simulink model "robotarm_A12"  (R2018b)
settings: Solver=FixedStepAuto  StartTime=0.0  StopTime=options.T_train  RelTol=1e-3  AbsTol=1e-6
undefined symbols (not defined in the file or in its folder): options
libraries: neural x132, simulink x2
(part 4 of 6)

== system robotarm_A12/NN/Layer 3/Delays 1 ==
  "p{3}" : Inport  PortDimensions=30
      mask Display: e = 0.06;c1 = [120 230 180]/255;c2 = ([120 230 180]+0)/(256+128);c3 = ([120 230 180]+128)/(256+128);patch([0 1 1 0],[0 0 1 1],c1);patch([0 1 1 1-e 1-e 0+e],[0 0 1 1-e 0+e 0+e],c2);patch([0 0 1 1-e 0+e 0+e],[0 1 1 1-e 1-e 0+e],c3);plot([0 1 1 0 0],[0 0 1 1 0]);
  mux : Mux  Inputs=1
      mask Display: e = 0.06;c1 = [120 150 230]/255;c2 = ([120 150 230]+0)/383;c3 = ([120 150 230]+128)/383;patch([0 1 1 0],[0 0 1 1],c1);patch([0 1 1 1-e 1-e 0+e],[0 0 1 1-e 0+e 0+e],c2);patch([0 0 1 1-e 0+e 0+e],[0 1 1 1-e 1-e 0+e],c3);plot([0 1 1 0 0],[0 0 1 1 0]);disp('Mux')
  "pd{3,2}" : Outport
      mask Display: e = 0.06;c1 = [120 230 180]/255;c2 = ([120 230 180]+0)/(256+128);c3 = ([120 230 180]+128)/(256+128);patch([0 1 1 0],[0 0 1 1],c1);patch([0 1 1 1-e 1-e 0+e],[0 0 1 1-e 0+e 0+e],c2);patch([0 0 1 1-e 0+e 0+e],[0 1 1 1-e 1-e 0+e],c3);plot([0 1 1 0 0],[0 0 1 1 0]);
  wires:
  "p{3}"/1 -> mux/1
  mux/1 -> "pd{3,2}"/1

== system robotarm_A12/NN/Layer 3/LW{3,2} ==
  "ad{3,2}" : Inport  PortDimensions=30
      mask Display: e = 0.06;c1 = [120 230 180]/255;c2 = ([120 230 180]+0)/(256+128);c3 = ([120 230 180]+128)/(256+128);patch([0 1 1 0],[0 0 1 1],c1);patch([0 1 1 1-e 1-e 0+e],[0 0 1 1-e 0+e 0+e],c2);patch([0 0 1 1-e 0+e 0+e],[0 1 1 1-e 1-e 0+e],c3);plot([0 1 1 0 0],[0 0 1 1 0]);
  "IW{3,2}(1,:)'" : Constant  Value=[0.1383029503063844811716620597508153878152370452880859375;0.429487160451053229248685738639323972165584564208984375;0.18901620447590949947169747247244231402873992919921875;0.32165527306370889082387520829797722399234771728515625;0.74909838521993721283109834985225461423397064208984375;0.73436150614245665479984381818212568759918212890625;-0.210267559609641718765260520740412175655364990234375;0.1637201058574380141408255440182983875274658203125;-0.08239392709912425616369802128247101791203022003173828125;-0.04209806064912581524684043188244686461985111236572265625;0.483612857722291622497579055561800487339496612548828125;-0.69853138032835115911467482874286361038684844970703125;0.366730507337538147449862435678369365632534027099609375;-0.1640502606970858090473797119557275436818599700927734375;0.203789426049731436929590699946857057511806488037109375;-0.08845604284062158484402971225790679454803466796875;0.57150676187570603747900577218388207256793975830078125;-0.51642895032712077263425953788100741803646087646484375;-0.2075569267144057594709494196649757213890552520751953125;0.1470866703039565293043011706686229445040225982666015625;-0.06293559925108438424246060094446875154972076416015625;0.6015475040548217133817843205179087817668914794921875;-0.2812003145211889876264876875211484730243682861328125;0.2088923518804825241179656813983456231653690338134765625;0.03580286806883258010625326051012962125241756439208984375;0.07831736039607979649179725356589187867939472198486328125;-0.1480431710605027983973513983073644340038299560546875;-0.53074776826549363573093387458357028663158416748046875;-0.07013101789848652511949467225349508225917816162109375;-0.39005646743948896304488016539835371077060699462890625]
      mask Display: e = 0.06;c1 = [120 150 230]/255;c2 = ([120 150 230]+0)/383;c3 = ([120 150 230]+128)/383;patch([0 1 1 0],[0 0 1 1],c1);patch([0 1 1 1-e 1-e 0+e],[0 0 1 1-e 0+e 0+e],c2);patch([0 0 1 1-e 0+e 0+e],[0 1 1 1-e 1-e 0+e],c3);plot([0 1 1 0 0],[0 0 1 1 0]);disp('weights');
  Mux : Mux  Inputs=1
      mask Display: e = 0.06;c1 = [120 150 230]/255;c2 = ([120 150 230]+0)/383;c3 = ([120 150 230]+128)/383;patch([0 1 1 0],[0 0 1 1],c1);patch([0 1 1 1-e 1-e 0+e],[0 0 1 1-e 0+e 0+e],c2);patch([0 0 1 1-e 0+e 0+e],[0 1 1 1-e 1-e 0+e],c3);plot([0 1 1 0 0],[0 0 1 1 0]);disp('Mux');
  dotprod1 : neural/Weight Functions/dotprod
  "lz{3,2}" : Outport
      mask Display: e = 0.06;c1 = [120 230 180]/255;c2 = ([120 230 180]+0)/(256+128);c3 = ([120 230 180]+128)/(256+128);patch([0 1 1 0],[0 0 1 1],c1);patch([0 1 1 1-e 1-e 0+e],[0 0 1 1-e 0+e 0+e],c2);patch([0 0 1 1-e 0+e 0+e],[0 1 1 1-e 1-e 0+e],c3);plot([0 1 1 0 0],[0 0 1 1 0]);
  wires:
  "IW{3,2}(1,:)'"/1 -> dotprod1/1
  "ad{3,2}"/1 -> dotprod1/2
  dotprod1/1 -> Mux/1
  Mux/1 -> "lz{3,2}"/1

== system robotarm_A12/NN_cex_1/Layer 1/Delays 1 ==
  "p{1}" : Inport  PortDimensions=10
      mask Display: e = 0.06;c1 = [120 230 180]/255;c2 = ([120 230 180]+0)/(256+128);c3 = ([120 230 180]+128)/(256+128);patch([0 1 1 0],[0 0 1 1],c1);patch([0 1 1 1-e 1-e 0+e],[0 0 1 1-e 0+e 0+e],c2);patch([0 0 1 1-e 0+e 0+e],[0 1 1 1-e 1-e 0+e],c3);plot([0 1 1 0 0],[0 0 1 1 0]);
  mux : Mux  Inputs=1
      mask Display: e = 0.06;c1 = [120 150 230]/255;c2 = ([120 150 230]+0)/383;c3 = ([120 150 230]+128)/383;patch([0 1 1 0],[0 0 1 1],c1);patch([0 1 1 1-e 1-e 0+e],[0 0 1 1-e 0+e 0+e],c2);patch([0 0 1 1-e 0+e 0+e],[0 1 1 1-e 1-e 0+e],c3);plot([0 1 1 0 0],[0 0 1 1 0]);disp('Mux')
  "pd{1,1}" : Outport
      mask Display: e = 0.06;c1 = [120 230 180]/255;c2 = ([120 230 180]+0)/(256+128);c3 = ([120 230 180]+128)/(256+128);patch([0 1 1 0],[0 0 1 1],c1);patch([0 1 1 1-e 1-e 0+e],[0 0 1 1-e 0+e 0+e],c2);patch([0 0 1 1-e 0+e 0+e],[0 1 1 1-e 1-e 0+e],c3);plot([0 1 1 0 0],[0 0 1 1 0]);
  wires:
  "p{1}"/1 -> mux/1
  mux/1 -> "pd{1,1}"/1

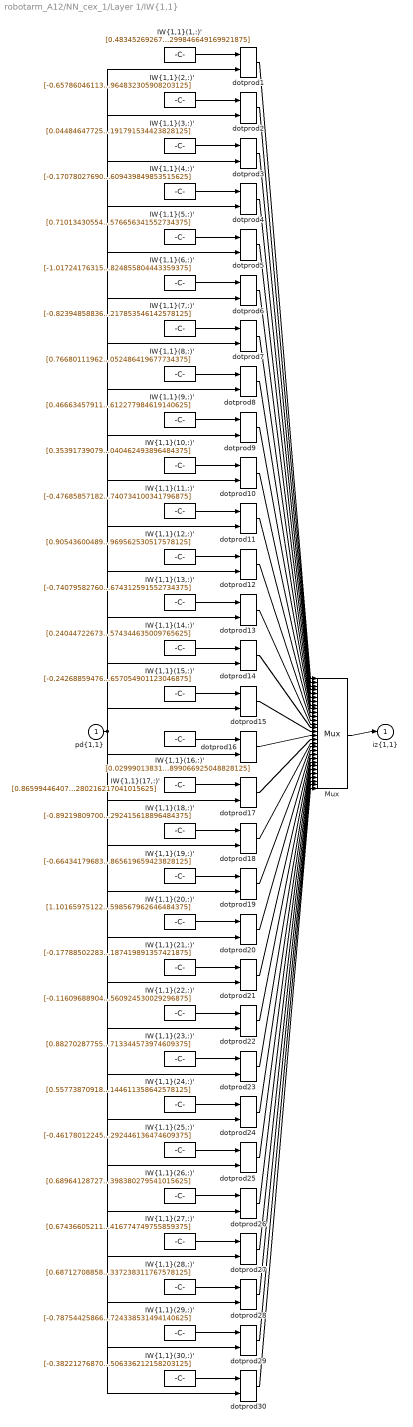
== system robotarm_A12/NN_cex_1/Layer 1/IW{1,1} ==
  "pd{1,1}" : Inport  PortDimensions=10
      mask Display: e = 0.06;c1 = [120 230 180]/255;c2 = ([120 230 180]+0)/(256+128);c3 = ([120 230 180]+128)/(256+128);patch([0 1 1 0],[0 0 1 1],c1);patch([0 1 1 1-e 1-e 0+e],[0 0 1 1-e 0+e 0+e],c2);patch([0 0 1 1-e 0+e 0+e],[0 1 1 1-e 1-e 0+e],c3);plot([0 1 1 0 0],[0 0 1 1 0]);
  "IW{1,1}(1,:)'" : Constant  Value=[0.4834526926789930456607180531136691570281982421875;-0.72644020956216104334401961750700138509273529052734375;0.6324505417251931049804625217802822589874267578125;-0.479360089533674316175648755233851261436939239501953125;0.62401522634030126557291850986075587570667266845703125;-0.32351142921760545068110559441265650093555450439453125;0.6698035013946872506807039826526306569576263427734375;-0.7690799010562889836961630862788297235965728759765625;-0.48612975307962502657943559825071133673191070556640625;-0.7473148686759862879824822812224738299846649169921875]
      mask Display: e = 0.06;c1 = [120 150 230]/255;c2 = ([120 150 230]+0)/383;c3 = ([120 150 230]+128)/383;patch([0 1 1 0],[0 0 1 1],c1);patch([0 1 1 1-e 1-e 0+e],[0 0 1 1-e 0+e 0+e],c2);patch([0 0 1 1-e 0+e 0+e],[0 1 1 1-e 1-e 0+e],c3);plot([0 1 1 0 0],[0 0 1 1 0]);disp('Weights');
  "IW{1,1}(10,:)'" : Constant  Value=[0.35391739079272321877311924254172481596469879150390625;0.95859782781468816370562535666977055370807647705078125;-0.54394161025246956508993889656267128884792327880859375;-0.150509093587718023599109073984436690807342529296875;-0.05447173836255088386071321338022244162857532501220703125;-0.364979095227050021055248407719773240387439727783203125;-0.788365061749647821898179245181381702423095703125;0.89626312931742824208214415193651802837848663330078125;0.604478218580114745606124415644444525241851806640625;-0.26236130241610611246727557954727672040462493896484375]
      mask Display: e = 0.06;c1 = [120 150 230]/255;c2 = ([120 150 230]+0)/383;c3 = ([120 150 230]+128)/383;patch([0 1 1 0],[0 0 1 1],c1);patch([0 1 1 1-e 1-e 0+e],[0 0 1 1-e 0+e 0+e],c2);patch([0 0 1 1-e 0+e 0+e],[0 1 1 1-e 1-e 0+e],c3);plot([0 1 1 0 0],[0 0 1 1 0]);disp('Weights');
  "IW{1,1}(11,:)'" : Constant  Value=[-0.4768585718260525130318683295627124607563018798828125;0.53555234975278853681857071933336555957794189453125;0.89898701204696662703241827330202795565128326416015625;0.517185573669362685933492684853263199329376220703125;-0.260990920148942595613306139057385735213756561279296875;-0.28998745558328453686414150070049799978733062744140625;-0.060061668087112864145016288830447592772543430328369140625;0.97511951323132206592703141723177395761013031005859375;0.63747862192401871794800172210671007633209228515625;-0.472832948738687530720881113666109740734100341796875]
      mask Display: e = 0.06;c1 = [120 150 230]/255;c2 = ([120 150 230]+0)/383;c3 = ([120 150 230]+128)/383;patch([0 1 1 0],[0 0 1 1],c1);patch([0 1 1 1-e 1-e 0+e],[0 0 1 1-e 0+e 0+e],c2);patch([0 0 1 1-e 0+e 0+e],[0 1 1 1-e 1-e 0+e],c3);plot([0 1 1 0 0],[0 0 1 1 0]);disp('Weights');
  "IW{1,1}(12,:)'" : Constant  Value=[0.90543600489521602892040164078935049474239349365234375;-1.183316184409171523128634362365119159221649169921875;0.80202518627175489740466218790970742702484130859375;0.00563310355029791355596646695857998565770685672760009765625;-0.2095477186078738285335276714249630458652973175048828125;0.213186578922721581275112612274824641644954681396484375;-0.417835039130007801499999686711817048490047454833984375;0.50032007982358150943724695025593973696231842041015625;0.5196382528120120358750000377767719328403472900390625;0.2418631247768887881921529015016858465969562530517578125]
      mask Display: e = 0.06;c1 = [120 150 230]/255;c2 = ([120 150 230]+0)/383;c3 = ([120 150 230]+128)/383;patch([0 1 1 0],[0 0 1 1],c1);patch([0 1 1 1-e 1-e 0+e],[0 0 1 1-e 0+e 0+e],c2);patch([0 0 1 1-e 0+e 0+e],[0 1 1 1-e 1-e 0+e],c3);plot([0 1 1 0 0],[0 0 1 1 0]);disp('Weights');
  "IW{1,1}(13,:)'" : Constant  Value=[-0.7407958276083366211395286882179789245128631591796875;-0.374173190683332268502425677070277743041515350341796875;-0.321859543990112906275413706680410541594028472900390625;0.053948177889655467287521872776778764091432094573974609375;-0.14745174018063400556144415531889535486698150634765625;-0.3043505897038809582255680652451701462268829345703125;-0.80965898869272479032588307745754718780517578125;0.610047747060808998043057727045379579067230224609375;-1.0123879702520695023082453189999796450138092041015625;-0.495161617801435249841546237803413532674312591552734375]
      mask Display: e = 0.06;c1 = [120 150 230]/255;c2 = ([120 150 230]+0)/383;c3 = ([120 150 230]+128)/383;patch([0 1 1 0],[0 0 1 1],c1);patch([0 1 1 1-e 1-e 0+e],[0 0 1 1-e 0+e 0+e],c2);patch([0 0 1 1-e 0+e 0+e],[0 1 1 1-e 1-e 0+e],c3);plot([0 1 1 0 0],[0 0 1 1 0]);disp('Weights');
  "IW{1,1}(14,:)'" : Constant  Value=[0.2404472267346937364163039774211938492953777313232421875;-0.005189758779571979931122260865095086046494543552398681640625;-0.498890641200198547977606722270138561725616455078125;0.70578607016098071635923361100140027701854705810546875;0.9057578305132747420458372289431281387805938720703125;-0.84934340490121140732071580714546144008636474609375;0.56837415725882645123334668824099935591220855712890625;-0.425752812183665785283892546431161463260650634765625;0.2222530086668008941774843378880177624523639678955078125;-0.15659255741849043008784292396740056574344635009765625]
      mask Display: e = 0.06;c1 = [120 150 230]/255;c2 = ([120 150 230]+0)/383;c3 = ([120 150 230]+128)/383;patch([0 1 1 0],[0 0 1 1],c1);patch([0 1 1 1-e 1-e 0+e],[0 0 1 1-e 0+e 0+e],c2);patch([0 0 1 1-e 0+e 0+e],[0 1 1 1-e 1-e 0+e],c3);plot([0 1 1 0 0],[0 0 1 1 0]);disp('Weights');
  "IW{1,1}(15,:)'" : Constant  Value=[-0.242688594763704801327008908629068173468112945556640625;0.71303675833753288326732899804483167827129364013671875;-0.04581829615003095435010749270077212713658809661865234375;0.73090669216345538483636801174725405871868133544921875;-0.516705265909575217619931208901107311248779296875;-0.10918366751174475581809275581690599210560321807861328125;0.76112004039804481703157534866477362811565399169921875;0.6932713431960479955051823708345182240009307861328125;-0.601143910429225325486868314328603446483612060546875;0.1322996482211735436163024814959499053657054901123046875]
      mask Display: e = 0.06;c1 = [120 150 230]/255;c2 = ([120 150 230]+0)/383;c3 = ([120 150 230]+128)/383;patch([0 1 1 0],[0 0 1 1],c1);patch([0 1 1 1-e 1-e 0+e],[0 0 1 1-e 0+e 0+e],c2);patch([0 0 1 1-e 0+e 0+e],[0 1 1 1-e 1-e 0+e],c3);plot([0 1 1 0 0],[0 0 1 1 0]);disp('Weights');
  "IW{1,1}(16,:)'" : Constant  Value=[0.029990138318937147043907742727242293767631053924560546875;0.11800395311584231661239385857697925530374050140380859375;0.82635631882874271969541268845205195248126983642578125;0.5192188532350889840216723314370028674602508544921875;0.38169266081526165290682683917111717164516448974609375;0.260924489046415353232788447712664492428302764892578125;0.7092110509581732724626590425032190978527069091796875;-0.2291987651974617679062617980889626778662204742431640625;-0.303748109565343649141055948348366655409336090087890625;0.61273400263456168080011821075459010899066925048828125]
      mask Display: e = 0.06;c1 = [120 150 230]/255;c2 = ([120 150 230]+0)/383;c3 = ([120 150 230]+128)/383;patch([0 1 1 0],[0 0 1 1],c1);patch([0 1 1 1-e 1-e 0+e],[0 0 1 1-e 0+e 0+e],c2);patch([0 0 1 1-e 0+e 0+e],[0 1 1 1-e 1-e 0+e],c3);plot([0 1 1 0 0],[0 0 1 1 0]);disp('Weights');
  "IW{1,1}(17,:)'" : Constant  Value=[0.8659944640706960239384670785511843860149383544921875;-0.6907088326519044141349468191037885844707489013671875;0.94454462704665897998523860223940573632717132568359375;-0.281648660685572316264568826227332465350627899169921875;0.47123942988213018967513789903023280203342437744140625;-0.79221396257464216095200981726520694792270660400390625;0.2200724445485724434234953150735236704349517822265625;0.2264868951875262659267917797478730790317058563232421875;-0.624722025098265465459235201706178486347198486328125;-0.418974861193588399288501022965647280216217041015625]
      mask Display: e = 0.06;c1 = [120 150 230]/255;c2 = ([120 150 230]+0)/383;c3 = ([120 150 230]+128)/383;patch([0 1 1 0],[0 0 1 1],c1);patch([0 1 1 1-e 1-e 0+e],[0 0 1 1-e 0+e 0+e],c2);patch([0 0 1 1-e 0+e 0+e],[0 1 1 1-e 1-e 0+e],c3);plot([0 1 1 0 0],[0 0 1 1 0]);disp('Weights');
  "IW{1,1}(18,:)'" : Constant  Value=[-0.8921980970068263960826016045757569372653961181640625;0.435199722097781294127827322881785221397876739501953125;-0.47382307465057704742861233171424828469753265380859375;-0.2077962998418919349230549187268479727208614349365234375;-0.1933921332739222676000423462028265930712223052978515625;-0.85931626506183800273674933123402297496795654296875;0.1950641592492608766828965372042148374021053314208984375;-0.1634953527516685711784560908199637196958065032958984375;-1.0122356572500341709286431068903766572475433349609375;-0.36320496498435816956629196283756755292415618896484375]
      mask Display: e = 0.06;c1 = [120 150 230]/255;c2 = ([120 150 230]+0)/383;c3 = ([120 150 230]+128)/383;patch([0 1 1 0],[0 0 1 1],c1);patch([0 1 1 1-e 1-e 0+e],[0 0 1 1-e 0+e 0+e],c2);patch([0 0 1 1-e 0+e 0+e],[0 1 1 1-e 1-e 0+e],c3);plot([0 1 1 0 0],[0 0 1 1 0]);disp('Weights');
  "IW{1,1}(19,:)'" : Constant  Value=[-0.66434179683580174557988584638223983347415924072265625;-0.42089894869251798237286266157752834260463714599609375;-0.155210098575526089792475659123738296329975128173828125;-0.57605400909988724311716623560641892254352569580078125;-0.5653615632923507661189432838000357151031494140625;-0.232282623120897369073389882032643072307109832763671875;0.75219064149188230583575887067127041518688201904296875;-0.471684135048713371052286902340711094439029693603515625;0.50962675577361327139414015618967823684215545654296875;0.32041852953757754551844527668436057865619659423828125]
      mask Display: e = 0.06;c1 = [120 150 230]/255;c2 = ([120 150 230]+0)/383;c3 = ([120 150 230]+128)/383;patch([0 1 1 0],[0 0 1 1],c1);patch([0 1 1 1-e 1-e 0+e],[0 0 1 1-e 0+e 0+e],c2);patch([0 0 1 1-e 0+e 0+e],[0 1 1 1-e 1-e 0+e],c3);plot([0 1 1 0 0],[0 0 1 1 0]);disp('Weights');
  "IW{1,1}(2,:)'" : Constant  Value=[-0.65786046113623719566732006569509394466876983642578125;-0.77256588266731684999655271894880570471286773681640625;0.56987155006092293785258107163826934993267059326171875;0.339750022138902263435511486022733151912689208984375;0.69641467418709901426865371831809170544147491455078125;-0.383167020142241743219102545481291599571704864501953125;1.0457628593329217903118433241616003215312957763671875;-0.490609642189974215487069386654184199869632720947265625;-0.42176619449435370778900278310175053775310516357421875;-0.07713472106713521736498506697898847050964832305908203125]
      mask Display: e = 0.06;c1 = [120 150 230]/255;c2 = ([120 150 230]+0)/383;c3 = ([120 150 230]+128)/383;patch([0 1 1 0],[0 0 1 1],c1);patch([0 1 1 1-e 1-e 0+e],[0 0 1 1-e 0+e 0+e],c2);patch([0 0 1 1-e 0+e 0+e],[0 1 1 1-e 1-e 0+e],c3);plot([0 1 1 0 0],[0 0 1 1 0]);disp('Weights');
  "IW{1,1}(20,:)'" : Constant  Value=[1.1016597512253467616716307020396925508975982666015625;-0.55507308593904891580450566834770143032073974609375;0.11880036289366917301446591181957046501338481903076171875;-0.496305403561088709363247062356094829738140106201171875;-0.152309479128132474468060308936401270329952239990234375;0.83277148857905902712417400834965519607067108154296875;0.0577009666156788891822060350023093633353710174560546875;-0.339001237191361159961644489158061333000659942626953125;0.1666252157714354920070576326907030306756496429443359375;0.64600906337637853393829345804988406598567962646484375]
      mask Display: e = 0.06;c1 = [120 150 230]/255;c2 = ([120 150 230]+0)/383;c3 = ([120 150 230]+128)/383;patch([0 1 1 0],[0 0 1 1],c1);patch([0 1 1 1-e 1-e 0+e],[0 0 1 1-e 0+e 0+e],c2);patch([0 0 1 1-e 0+e 0+e],[0 1 1 1-e 1-e 0+e],c3);plot([0 1 1 0 0],[0 0 1 1 0]);disp('Weights');
  "IW{1,1}(21,:)'" : Constant  Value=[-0.1778850228348457240823421443565166555345058441162109375;-0.8231162386450050494346442064852453768253326416015625;0.82444320496735468140059310826472938060760498046875;0.07408990623263796149178261885026586242020130157470703125;0.5374113301635035089276470898767001926898956298828125;-0.449339591780794578301794217622955329716205596923828125;0.54538474460031494128742224347661249339580535888671875;0.13097128114349565475293957206304185092449188232421875;-0.69134538818886770439320343939471058547496795654296875;-0.72425734763447813246983741919393651187419891357421875]
      mask Display: e = 0.06;c1 = [120 150 230]/255;c2 = ([120 150 230]+0)/383;c3 = ([120 150 230]+128)/383;patch([0 1 1 0],[0 0 1 1],c1);patch([0 1 1 1-e 1-e 0+e],[0 0 1 1-e 0+e 0+e],c2);patch([0 0 1 1-e 0+e 0+e],[0 1 1 1-e 1-e 0+e],c3);plot([0 1 1 0 0],[0 0 1 1 0]);disp('Weights');
  "IW{1,1}(22,:)'" : Constant  Value=[-0.116096889043422912823899650902603752911090850830078125;0.8650782780629995283305788689176551997661590576171875;-0.95548476670328208459892493920051492750644683837890625;-0.305761347228730884229008779584546573460102081298828125;-0.273437745508399887572892339449026621878147125244140625;-0.665330595028158722215039233560673892498016357421875;0.828673165748145645892464017379097640514373779296875;-0.5116471905218038518370349265751428902149200439453125;-0.1476817579101468991265022623338154517114162445068359375;0.62081089404955125399254711737739853560924530029296875]
      mask Display: e = 0.06;c1 = [120 150 230]/255;c2 = ([120 150 230]+0)/383;c3 = ([120 150 230]+128)/383;patch([0 1 1 0],[0 0 1 1],c1);patch([0 1 1 1-e 1-e 0+e],[0 0 1 1-e 0+e 0+e],c2);patch([0 0 1 1-e 0+e 0+e],[0 1 1 1-e 1-e 0+e],c3);plot([0 1 1 0 0],[0 0 1 1 0]);disp('Weights');
  "IW{1,1}(23,:)'" : Constant  Value=[0.8827028775551177819380654909764416515827178955078125;0.2182201298955653567812618121024570427834987640380859375;-0.338355242198717098833782301881001330912113189697265625;0.4519214532903192971247108289389871060848236083984375;-0.299496443749006413526103642652742564678192138671875;-0.5611895294678130863275100637110881507396697998046875;0.0695757552620342722971003013299196027219295501708984375;-0.054649848724784545750399189500967622734606266021728515625;-0.333246012112561496021356788332923315465450286865234375;0.88441095482990339515794175895280204713344573974609375]
      mask Display: e = 0.06;c1 = [120 150 230]/255;c2 = ([120 150 230]+0)/383;c3 = ([120 150 230]+128)/383;patch([0 1 1 0],[0 0 1 1],c1);patch([0 1 1 1-e 1-e 0+e],[0 0 1 1-e 0+e 0+e],c2);patch([0 0 1 1-e 0+e 0+e],[0 1 1 1-e 1-e 0+e],c3);plot([0 1 1 0 0],[0 0 1 1 0]);disp('Weights');
  "IW{1,1}(24,:)'" : Constant  Value=[0.55773870918581158750981785487965680658817291259765625;0.1623167340065563568618500767115619964897632598876953125;0.438168275413182650712684562677168287336826324462890625;-1.32325043302354838914425272378139197826385498046875;-0.1782573157111801975815978948958218097686767578125;0.27895979933631676050964642854523845016956329345703125;-0.2278922769292026639931236786651425063610076904296875;0.39819142600306556278866310094599612057209014892578125;0.11298478527026246942543963314165011979639530181884765625;-0.7048134209472813882513264616136439144611358642578125]
      mask Display: e = 0.06;c1 = [120 150 230]/255;c2 = ([120 150 230]+0)/383;c3 = ([120 150 230]+128)/383;patch([0 1 1 0],[0 0 1 1],c1);patch([0 1 1 1-e 1-e 0+e],[0 0 1 1-e 0+e 0+e],c2);patch([0 0 1 1-e 0+e 0+e],[0 1 1 1-e 1-e 0+e],c3);plot([0 1 1 0 0],[0 0 1 1 0]);disp('Weights');
  "IW{1,1}(25,:)'" : Constant  Value=[-0.461780122459949871061013482176349498331546783447265625;-0.64127008235733173879822288654395379126071929931640625;0.49572317787502895303219929701299406588077545166015625;0.53585608341899959583543022745288908481597900390625;-0.017168922521098105293813063099150895141065120697021484375;0.89099790557429658921506643309840001165866851806640625;-0.44690350535643463825152821300434879958629608154296875;0.415739848583360827039001605953671969473361968994140625;-0.63559312870218398483501687223906628787517547607421875;0.285175255516433912017504326286143623292446136474609375]
      mask Display: e = 0.06;c1 = [120 150 230]/255;c2 = ([120 150 230]+0)/383;c3 = ([120 150 230]+128)/383;patch([0 1 1 0],[0 0 1 1],c1);patch([0 1 1 1-e 1-e 0+e],[0 0 1 1-e 0+e 0+e],c2);patch([0 0 1 1-e 0+e 0+e],[0 1 1 1-e 1-e 0+e],c3);plot([0 1 1 0 0],[0 0 1 1 0]);disp('Weights');
  "IW{1,1}(26,:)'" : Constant  Value=[0.68964128727552054254346103334682993590831756591796875;-0.73834912383953288372850920495693571865558624267578125;0.1637316570409002025598965701647102832794189453125;-0.43330206176185404043366133919334970414638519287109375;-1.06444251686522495248254926991648972034454345703125;0.58403490056535900531997640428016893565654754638671875;0.83733725961995963960049493834958411753177642822265625;-0.06427552440278620771163531344427610747516155242919921875;0.216857387087115716095553352715796791017055511474609375;0.39975312907853377542011230616481043398380279541015625]
      mask Display: e = 0.06;c1 = [120 150 230]/255;c2 = ([120 150 230]+0)/383;c3 = ([120 150 230]+128)/383;patch([0 1 1 0],[0 0 1 1],c1);patch([0 1 1 1-e 1-e 0+e],[0 0 1 1-e 0+e 0+e],c2);patch([0 0 1 1-e 0+e 0+e],[0 1 1 1-e 1-e 0+e],c3);plot([0 1 1 0 0],[0 0 1 1 0]);disp('Weights');
  "IW{1,1}(27,:)'" : Constant  Value=[0.6743660521128875817709058537730015814304351806640625;0.1674897261703397755017164172386401332914829254150390625;-0.260164955623930993500181330091436393558979034423828125;0.822915206644074803676858209655620157718658447265625;0.184372473394916747135852119754417799413204193115234375;0.1505134107924354369689723398550995625555515289306640625;-0.77076982205334321207601533387787640094757080078125;0.70220734276975471654935745391412638127803802490234375;0.481173293810763180733403032718342728912830352783203125;-0.88802732306203324696980416774749755859375]
      mask Display: e = 0.06;c1 = [120 150 230]/255;c2 = ([120 150 230]+0)/383;c3 = ([120 150 230]+128)/383;patch([0 1 1 0],[0 0 1 1],c1);patch([0 1 1 1-e 1-e 0+e],[0 0 1 1-e 0+e 0+e],c2);patch([0 0 1 1-e 0+e 0+e],[0 1 1 1-e 1-e 0+e],c3);plot([0 1 1 0 0],[0 0 1 1 0]);disp('Weights');
  "IW{1,1}(28,:)'" : Constant  Value=[0.68712708858233384479063943217624910175800323486328125;-0.66541022041782793561282005612156353890895843505859375;-0.394952835975215688080197651288472115993499755859375;0.332051651689891258456555078737437725067138671875;-0.82856097386912230806643719915882684290409088134765625;0.01816410281411696969744440366412163712084293365478515625;0.57251355549686400170372735374257899820804595947265625;0.71850346186628699651777196777402423322200775146484375;-0.533045535111253965254718423238955438137054443359375;-0.3771111188430673610838539389078505337238311767578125]
      mask Display: e = 0.06;c1 = [120 150 230]/255;c2 = ([120 150 230]+0)/383;c3 = ([120 150 230]+128)/383;patch([0 1 1 0],[0 0 1 1],c1);patch([0 1 1 1-e 1-e 0+e],[0 0 1 1-e 0+e 0+e],c2);patch([0 0 1 1-e 0+e 0+e],[0 1 1 1-e 1-e 0+e],c3);plot([0 1 1 0 0],[0 0 1 1 0]);disp('Weights');
  "IW{1,1}(29,:)'" : Constant  Value=[-0.7875442586601943961710503572248853743076324462890625;-0.54049475580268424579344355151988565921783447265625;0.874994303368197723358434814144857227802276611328125;0.580822164501316517970508357393555343151092529296875;0.01155276382962600913162365401376519002951681613922119140625;-0.76076298435945599596408328579855151474475860595703125;0.57246350445777094417820762828341685235500335693359375;-0.5181405023297365186607521536643616855144500732421875;0.300301675760051678398809826830984093248844146728515625;0.646514982582135022681768532493151724338531494140625]
      mask Display: e = 0.06;c1 = [120 150 230]/255;c2 = ([120 150 230]+0)/383;c3 = ([120 150 230]+128)/383;patch([0 1 1 0],[0 0 1 1],c1);patch([0 1 1 1-e 1-e 0+e],[0 0 1 1-e 0+e 0+e],c2);patch([0 0 1 1-e 0+e 0+e],[0 1 1 1-e 1-e 0+e],c3);plot([0 1 1 0 0],[0 0 1 1 0]);disp('Weights');
  "IW{1,1}(3,:)'" : Constant  Value=[0.044846477258794918696604980823394726030528545379638671875;0.794975187046314868410945564392022788524627685546875;-0.136735697072330963930397729200194589793682098388671875;0.04801385648509524928240210783769725821912288665771484375;0.177701353551733387536870623080176301300525665283203125;-0.82957030143161369917237379922880791127681732177734375;0.698647497206471346231637653545476496219635009765625;0.337609136454682323691400824827724136412143707275390625;0.5216390395504395538495145956403575837612152099609375;-0.589092867550946142074508315999992191791534423828125]
      mask Display: e = 0.06;c1 = [120 150 230]/255;c2 = ([120 150 230]+0)/383;c3 = ([120 150 230]+128)/383;patch([0 1 1 0],[0 0 1 1],c1);patch([0 1 1 1-e 1-e 0+e],[0 0 1 1-e 0+e 0+e],c2);patch([0 0 1 1-e 0+e 0+e],[0 1 1 1-e 1-e 0+e],c3);plot([0 1 1 0 0],[0 0 1 1 0]);disp('Weights');
  "IW{1,1}(30,:)'" : Constant  Value=[-0.382212768704402627850669205145095475018024444580078125;-0.74307772762406354427611177015933208167552947998046875;-0.96604381875815514835181829766952432692050933837890625;0.3634845636664871815213473382755182683467864990234375;-0.54122533071079648170353948444244451820850372314453125;-0.062620751482162340106896181168849579989910125732421875;-0.39842875602766680831479106927872635424137115478515625;0.298478388798536886650225596895324997603893280029296875;-0.76263710765213355013969476203783415257930755615234375;0.79380964581874036145592299362760968506336212158203125]
      mask Display: e = 0.06;c1 = [120 150 230]/255;c2 = ([120 150 230]+0)/383;c3 = ([120 150 230]+128)/383;patch([0 1 1 0],[0 0 1 1],c1);patch([0 1 1 1-e 1-e 0+e],[0 0 1 1-e 0+e 0+e],c2);patch([0 0 1 1-e 0+e 0+e],[0 1 1 1-e 1-e 0+e],c3);plot([0 1 1 0 0],[0 0 1 1 0]);disp('Weights');
  "IW{1,1}(4,:)'" : Constant  Value=[-0.1707802769072832849150955780714866705238819122314453125;-0.01412014037423006858340546187946529244072735309600830078125;0.1231328529920014125398353144191787578165531158447265625;0.31975044769631633112538793284329585731029510498046875;-0.44293953869965230207839113063528202474117279052734375;0.770644010674762736101683913148008286952972412109375;-0.230479014785789415586947370684356428682804107666015625;-0.7081006568464418560182593864738009870052337646484375;0.904952654231384823191319810575805604457855224609375;-1.0253737659838420004376757788122631609439849853515625]
      mask Display: e = 0.06;c1 = [120 150 230]/255;c2 = ([120 150 230]+0)/383;c3 = ([120 150 230]+128)/383;patch([0 1 1 0],[0 0 1 1],c1);patch([0 1 1 1-e 1-e 0+e],[0 0 1 1-e 0+e 0+e],c2);patch([0 0 1 1-e 0+e 0+e],[0 1 1 1-e 1-e 0+e],c3);plot([0 1 1 0 0],[0 0 1 1 0]);disp('Weights');
  "IW{1,1}(5,:)'" : Constant  Value=[0.710134305544150468136876952485181391239166259765625;-0.94089787939943902994599511657725088298320770263671875;0.28846596458657802752867382878321222960948944091796875;-0.2911628736779772186338277606409974396228790283203125;0.90967792520828982816283314605243504047393798828125;-0.362787948306247554075554262453806586563587188720703125;-0.50775442120664082690240093143074773252010345458984375;0.283871593429893154247878328533261083066463470458984375;-0.72296258765138821100748600656515918672084808349609375;0.487851855976706383355434581972076557576656341552734375]
      mask Display: e = 0.06;c1 = [120 150 230]/255;c2 = ([120 150 230]+0)/383;c3 = ([120 150 230]+128)/383;patch([0 1 1 0],[0 0 1 1],c1);patch([0 1 1 1-e 1-e 0+e],[0 0 1 1-e 0+e 0+e],c2);patch([0 0 1 1-e 0+e 0+e],[0 1 1 1-e 1-e 0+e],c3);plot([0 1 1 0 0],[0 0 1 1 0]);disp('Weights');
  "IW{1,1}(6,:)'" : Constant  Value=[-1.0172417631596297749041468705399893224239349365234375;0.60339893233243280246114181863958947360515594482421875;0.57240701753970280041272644666605629026889801025390625;-0.158092968679218903726990674840635620057582855224609375;-0.79666175002202932464712148430407978594303131103515625;-0.64151298364323039447043584004859440028667449951171875;0.1047002499193982194558572018650011159479618072509765625;-0.043645345270083089894708194833583547733724117279052734375;0.5861663917434043469256721436977386474609375;0.284327301808276755590298989773145876824855804443359375]
      mask Display: e = 0.06;c1 = [120 150 230]/255;c2 = ([120 150 230]+0)/383;c3 = ([120 150 230]+128)/383;patch([0 1 1 0],[0 0 1 1],c1);patch([0 1 1 1-e 1-e 0+e],[0 0 1 1-e 0+e 0+e],c2);patch([0 0 1 1-e 0+e 0+e],[0 1 1 1-e 1-e 0+e],c3);plot([0 1 1 0 0],[0 0 1 1 0]);disp('Weights');
  "IW{1,1}(7,:)'" : Constant  Value=[-0.82394858836690831882521024454035796225070953369140625;-0.1738404583501436395653882982514915056526660919189453125;0.049776878744683790423142255576749448664486408233642578125;-0.48410769343542259246504499969887547194957733154296875;-0.82677626282748029051816729406709782779216766357421875;-0.71012372572290949346296429212088696658611297607421875;0.54797935473956582708154883221141062676906585693359375;0.54282487246949917558680454021668992936611175537109375;0.57778721225832441188430266265640966594219207763671875;-0.108269514984206616237116804768447764217853546142578125]
      mask Display: e = 0.06;c1 = [120 150 230]/255;c2 = ([120 150 230]+0)/383;c3 = ([120 150 230]+128)/383;patch([0 1 1 0],[0 0 1 1],c1);patch([0 1 1 1-e 1-e 0+e],[0 0 1 1-e 0+e 0+e],c2);patch([0 0 1 1-e 0+e 0+e],[0 1 1 1-e 1-e 0+e],c3);plot([0 1 1 0 0],[0 0 1 1 0]);disp('Weights');
  "IW{1,1}(8,:)'" : Constant  Value=[0.7668011196207256130463747467729263007640838623046875;-0.9705819422182739852900112964562140405178070068359375;-0.594550256739938998151728810626082122325897216796875;0.78998111379925839425908407065435312688350677490234375;0.2417884805048096108492927669431082904338836669921875;-0.407673045493826158303107831670786254107952117919921875;0.374415596985115894934637026381096802651882171630859375;-0.74066956841357356466915007331408560276031494140625;0.52660097663042559901214190176688134670257568359375;0.1725047135584583113399048670544289052486419677734375]
      mask Display: e = 0.06;c1 = [120 150 230]/255;c2 = ([120 150 230]+0)/383;c3 = ([120 150 230]+128)/383;patch([0 1 1 0],[0 0 1 1],c1);patch([0 1 1 1-e 1-e 0+e],[0 0 1 1-e 0+e 0+e],c2);patch([0 0 1 1-e 0+e 0+e],[0 1 1 1-e 1-e 0+e],c3);plot([0 1 1 0 0],[0 0 1 1 0]);disp('Weights');
  "IW{1,1}(9,:)'" : Constant  Value=[0.466634579114610092975823363303788937628269195556640625;0.55493791872997022540658917932887561619281768798828125;-0.355632670353223601100722817136556841433048248291015625;-0.64444375836788048150793883905862458050251007080078125;-0.496587819718964429416274697359767742455005645751953125;1.000014913642893521483756558154709637165069580078125;-0.8667419735182539941575896591530181467533111572265625;0.09942209305355904913614750739725423045456409454345703125;-0.13364491312491910690596341737546026706695556640625;-0.7520270379888476242058459320105612277984619140625]
      mask Display: e = 0.06;c1 = [120 150 230]/255;c2 = ([120 150 230]+0)/383;c3 = ([120 150 230]+128)/383;patch([0 1 1 0],[0 0 1 1],c1);patch([0 1 1 1-e 1-e 0+e],[0 0 1 1-e 0+e 0+e],c2);patch([0 0 1 1-e 0+e 0+e],[0 1 1 1-e 1-e 0+e],c3);plot([0 1 1 0 0],[0 0 1 1 0]);disp('Weights');
  Mux : Mux  Inputs=30
      mask Display: e = 0.06;c1 = [120 150 230]/255;c2 = ([120 150 230]+0)/383;c3 = ([120 150 230]+128)/383;patch([0 1 1 0],[0 0 1 1],c1);patch([0 1 1 1-e 1-e 0+e],[0 0 1 1-e 0+e 0+e],c2);patch([0 0 1 1-e 0+e 0+e],[0 1 1 1-e 1-e 0+e],c3);plot([0 1 1 0 0],[0 0 1 1 0]);disp('Mux');
  dotprod{1..30} (30 alike) : neural/Weight Functions/dotprod
  "iz{1,1}" : Outport
      mask Display: e = 0.06;c1 = [120 230 180]/255;c2 = ([120 230 180]+0)/(256+128);c3 = ([120 230 180]+128)/(256+128);patch([0 1 1 0],[0 0 1 1],c1);patch([0 1 1 1-e 1-e 0+e],[0 0 1 1-e 0+e 0+e],c2);patch([0 0 1 1-e 0+e 0+e],[0 1 1 1-e 1-e 0+e],c3);plot([0 1 1 0 0],[0 0 1 1 0]);
  wires:
  "IW{1,1}(1,:)'"/1 -> dotprod1/1
  "pd{1,1}"/1 -> dotprod1/2, dotprod2/2, dotprod3/2, dotprod4/2, dotprod5/2, dotprod6/2, dotprod7/2, dotprod8/2, dotprod9/2, dotprod10/2, dotprod11/2, dotprod12/2, dotprod13/2, dotprod14/2, dotprod15/2, dotprod16/2, dotprod17/2, dotprod18/2, dotprod19/2, dotprod20/2, dotprod21/2, dotprod22/2, dotprod23/2, dotprod24/2, dotprod25/2, dotprod26/2, dotprod27/2, dotprod28/2, dotprod29/2, dotprod30/2
  dotprod1/1 -> Mux/1
  "IW{1,1}(2,:)'"/1 -> dotprod2/1
  dotprod2/1 -> Mux/2
  "IW{1,1}(3,:)'"/1 -> dotprod3/1
  dotprod3/1 -> Mux/3
  "IW{1,1}(4,:)'"/1 -> dotprod4/1
  dotprod4/1 -> Mux/4
  "IW{1,1}(5,:)'"/1 -> dotprod5/1
  dotprod5/1 -> Mux/5
  "IW{1,1}(6,:)'"/1 -> dotprod6/1
  dotprod6/1 -> Mux/6
  "IW{1,1}(7,:)'"/1 -> dotprod7/1
  dotprod7/1 -> Mux/7
  "IW{1,1}(8,:)'"/1 -> dotprod8/1
  dotprod8/1 -> Mux/8
  "IW{1,1}(9,:)'"/1 -> dotprod9/1
  dotprod9/1 -> Mux/9
  "IW{1,1}(10,:)'"/1 -> dotprod10/1
  dotprod10/1 -> Mux/10
  "IW{1,1}(11,:)'"/1 -> dotprod11/1
  dotprod11/1 -> Mux/11
  "IW{1,1}(12,:)'"/1 -> dotprod12/1
  dotprod12/1 -> Mux/12
  "IW{1,1}(13,:)'"/1 -> dotprod13/1
  dotprod13/1 -> Mux/13
  "IW{1,1}(14,:)'"/1 -> dotprod14/1
  dotprod14/1 -> Mux/14
  "IW{1,1}(15,:)'"/1 -> dotprod15/1
  dotprod15/1 -> Mux/15
  "IW{1,1}(16,:)'"/1 -> dotprod16/1
  dotprod16/1 -> Mux/16
  "IW{1,1}(17,:)'"/1 -> dotprod17/1
  dotprod17/1 -> Mux/17
  "IW{1,1}(18,:)'"/1 -> dotprod18/1
  dotprod18/1 -> Mux/18
  "IW{1,1}(19,:)'"/1 -> dotprod19/1
  dotprod19/1 -> Mux/19
  "IW{1,1}(20,:)'"/1 -> dotprod20/1
  dotprod20/1 -> Mux/20
  "IW{1,1}(21,:)'"/1 -> dotprod21/1
  dotprod21/1 -> Mux/21
  "IW{1,1}(22,:)'"/1 -> dotprod22/1
  dotprod22/1 -> Mux/22
  "IW{1,1}(23,:)'"/1 -> dotprod23/1
  dotprod23/1 -> Mux/23
  "IW{1,1}(24,:)'"/1 -> dotprod24/1
  dotprod24/1 -> Mux/24
  "IW{1,1}(25,:)'"/1 -> dotprod25/1
  dotprod25/1 -> Mux/25
  "IW{1,1}(26,:)'"/1 -> dotprod26/1
  dotprod26/1 -> Mux/26
  "IW{1,1}(27,:)'"/1 -> dotprod27/1
  dotprod27/1 -> Mux/27
  "IW{1,1}(28,:)'"/1 -> dotprod28/1
  dotprod28/1 -> Mux/28
  "IW{1,1}(29,:)'"/1 -> dotprod29/1
  dotprod29/1 -> Mux/29
  "IW{1,1}(30,:)'"/1 -> dotprod30/1
  dotprod30/1 -> Mux/30
  Mux/1 -> "iz{1,1}"/1

== system robotarm_A12/NN_cex_1/Layer 2/Delays 1 ==
  "p{2}" : Inport  PortDimensions=30
      mask Display: e = 0.06;c1 = [120 230 180]/255;c2 = ([120 230 180]+0)/(256+128);c3 = ([120 230 180]+128)/(256+128);patch([0 1 1 0],[0 0 1 1],c1);patch([0 1 1 1-e 1-e 0+e],[0 0 1 1-e 0+e 0+e],c2);patch([0 0 1 1-e 0+e 0+e],[0 1 1 1-e 1-e 0+e],c3);plot([0 1 1 0 0],[0 0 1 1 0]);
  mux : Mux  Inputs=1
      mask Display: e = 0.06;c1 = [120 150 230]/255;c2 = ([120 150 230]+0)/383;c3 = ([120 150 230]+128)/383;patch([0 1 1 0],[0 0 1 1],c1);patch([0 1 1 1-e 1-e 0+e],[0 0 1 1-e 0+e 0+e],c2);patch([0 0 1 1-e 0+e 0+e],[0 1 1 1-e 1-e 0+e],c3);plot([0 1 1 0 0],[0 0 1 1 0]);disp('Mux')
  "pd{2,1}" : Outport
      mask Display: e = 0.06;c1 = [120 230 180]/255;c2 = ([120 230 180]+0)/(256+128);c3 = ([120 230 180]+128)/(256+128);patch([0 1 1 0],[0 0 1 1],c1);patch([0 1 1 1-e 1-e 0+e],[0 0 1 1-e 0+e 0+e],c2);patch([0 0 1 1-e 0+e 0+e],[0 1 1 1-e 1-e 0+e],c3);plot([0 1 1 0 0],[0 0 1 1 0]);
  wires:
  "p{2}"/1 -> mux/1
  mux/1 -> "pd{2,1}"/1
